simulink model "test_climate"  (R2021a)
settings: Solver=VariableStepAuto  StartTime=0.0  StopTime=1  RelTol=1e-3
values from neighbouring files (symbols this model uses):
  ic_test01 = struct(ic_test01)    [test_climate_script.m]
  params_test01_st = struct(params_test01)    [test_climate_script.m]
libraries: HORTISIM x1
settings Model: Creator=djoroya  LastModifiedBy=djoroya

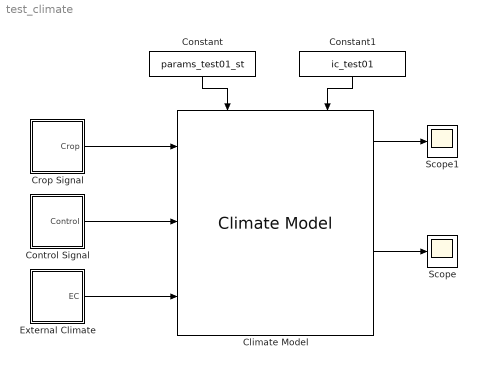
== system test_climate ==
  Climate Model : HORTISIM/Climate/Climate Model  SystemSampleTime=-1  VariantActivationTime=update diagram  Latency=0  AutoFrameSizeCalculation=off
      settings: SourceProductName=Horti Simulator  PortSchema="{\"entries\":[{\"content\":{\"sides\":[{\"content\":{\"connectorIds\":[\"In1\",\"In2\",\"In3\"]},\"type\":\"ConnectorPlacement.EquallySpacedRectSide\",\"uuid\":\"fdbdd374-8b10-44b2-b920-7342db253c10\"},{\"content\":{\"connectorIds\":[\"Out1\",\"Out2\",\"Out3\",\"Out4\"],\"side\":\"RIGHT\"},\"type\":\"ConnectorPlacement.EquallySpacedRectSide\",\"uuid\":\"ebf2dedb-5cad-43a3-941f-9afbcfcd0cc5\"},{\"content\":{\"connectorIds\":[\"In4\",\"In5\"],\"side\":\"TOP\"},\"type\":\"ConnectorPlacement.EquallySpacedRectSide\",\"uuid\":\"a5212d8e-fb05-4e50-b842-5c88822e5573\"},{\"content\":{\"connectorIds\":[],\"side\":\"BOTTOM\"},\"type\":\"ConnectorPlacement.EquallySpacedRectSide\",\"uuid\":\"6b5ac995-fd1e-4ed0-bd38-d85fddb17fbc\"}]},\"type\":\"ConnectorPlacement.EquallySpacedConnector\",\"uuid\":\"edcbb998-e937-4beb-a6bf-2c8d0dfc06bf\"}],\"packageUris\":[\"http://schema.mathworks.com/mf0/Connector/R2020b\"],\"version\":\"1.0\"}"
  Constant : Constant  Value=params_test01_st  OutDataTypeStr=Bus: slBus1
  Constant1 : Constant  Value=ic_test01  OutDataTypeStr=Bus: slBus2
  Control Signal : Subsystem
  Crop Signal : Subsystem
  External Climate : Subsystem
  Scope : Scope
  Scope1 : Scope
  wires:
  Crop Signal/1(Crop) -> Climate Model/1
  External Climate/1(EC) -> Climate Model/3
  Control Signal/1(Control) -> Climate Model/2
  Constant/1 -> Climate Model/4
  Constant1/1 -> Climate Model/5
  Climate Model/3 -> Scope/1
  Climate Model/1 -> Scope1/1

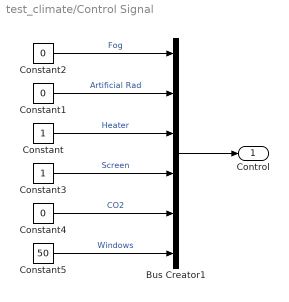
== system test_climate/Control Signal ==
  Bus Creator1 : BusCreator  Inputs=6
  Constant : Constant
  Constant1 : Constant  Value=0
  Constant2 : Constant  Value=0
  Constant3 : Constant
  Constant4 : Constant  Value=0
  Constant5 : Constant  Value=50
  Control : Outport
  wires:
  Constant/1 -> Bus Creator1/3  "Heater"
  Bus Creator1/1 -> Control/1
  Constant2/1 -> Bus Creator1/1  "Fog"
  Constant1/1 -> Bus Creator1/2  "Artificial Rad"
  Constant3/1 -> Bus Creator1/4  "Screen"
  Constant4/1 -> Bus Creator1/5  "CO2"
  Constant5/1 -> Bus Creator1/6  "Windows"

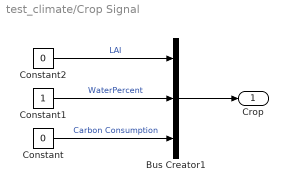
== system test_climate/Crop Signal ==
  Bus Creator1 : BusCreator  Inputs=3
  Constant : Constant  Value=0
  Constant1 : Constant
  Constant2 : Constant  Value=0
  Crop : Outport
  wires:
  Constant/1 -> Bus Creator1/3  "Carbon Consumption"
  Bus Creator1/1 -> Crop/1
  Constant2/1 -> Bus Creator1/1  "LAI"
  Constant1/1 -> Bus Creator1/2  "WaterPercent"

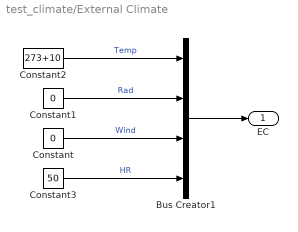
== system test_climate/External Climate ==
  Bus Creator1 : BusCreator  Inputs=4
  Constant : Constant  Value=0
  Constant1 : Constant  Value=0
  Constant2 : Constant  Value=273+10
  Constant3 : Constant  Value=50
  EC : Outport
  wires:
  Constant/1 -> Bus Creator1/3  "Wind"
  Bus Creator1/1 -> EC/1
  Constant2/1 -> Bus Creator1/1  "Temp"
  Constant1/1 -> Bus Creator1/2  "Rad"
  Constant3/1 -> Bus Creator1/4  "HR"
